simulink model "Extended_Kalman_Filter_Simulink_Example"  (R2024b)
settings: Solver=VariableStepAuto  StartTime=0.0  StopTime=20  RelTol=1e-3
libraries: simulink x5
settings Model: Creator=mulusoy  LastModifiedBy=fouca
settings SolverCC: AlgebraicLoopSolver=TrustRegion
settings DataIOCC: ReturnWorkspaceOutputs=off
settings OptimizationCC: BlockReduction=off  DefaultParameterBehavior=Inlined  ExpressionFolding=off  PassReuseOutputArgsAs=Individual arguments  EfficientTunableParamExpr=on
settings DebuggingCC: ParameterTunabilityLossMsg=error  ArithmeticOperatorsInVariantConditions=warning
settings ModelReferenceCC: EnableRefExpFcnMdlSchedulingChecks=on
settings SFSimCC: SimUseLocalCustomCode=off  MATLABDynamicMemAlloc=off  CustomCodeUndefinedFunction=UseInterfaceOnly
settings RTWCC: Description=Embedded Coder  SystemTargetFile=ert.tlc  GenCodeOnly=on  TemplateMakefile=ert_default_tmf  GenerateReport=on  RTWUseLocalCustomCode=off  IncludeHyperlinkInReport=on  LaunchReport=on  GenerateTraceInfo=on  GenerateTraceReport=on  GenerateTraceReportSl=on  GenerateTraceReportSf=on  GenerateTraceReportEml=on  GPUComputeCapability=3.5
settings CodeAppCC: ForceParamTrailComments=on  IgnoreCustomStorageClasses=off  OperatorAnnotations=on  SimulinkDataObjDesc=on  SFDataObjDesc=on  MATLABFcnDesc=on  InsertBlockDesc=on  StateflowObjectComments=on  MATLABSourceComments=on  EnableCustomComments=on  InlinedPrmAccess=Macros  ReqsInCode=on
settings ERTTargetCC: TargetLangStandard=C99 (ISO)  GenerateSampleERTMain=on  ERTCustomFileTemplate=example_file_process.tlc  ConvertIfToSwitch=off  DynamicArrayContainerType=coder::array
settings DiagnosticsConfigSet: SimMechanicsInvalidVisualProperty=none  SimMechanicsCrossSectionNullEdge=none  SimMechanicsUnconnectedFramePorts=none  SimMechanicsUnconnectedGeometryPorts=none  SimMechanicsRedundantBlock=none  SimMechanicsConflictingReferenceFrames=none  SimMechanicsUnsatisfiedHighPriorityTargets=none
settings ExplorerConfigSet: InternalSimMechanicsExplorerSettings="<ExplorerConfiguration><canonicalview>aerospace</canonicalview><AnimationSetting><BasePlaybackSpeed>1.0</BasePlaybackSpeed><PlaybackSpeedFactor>1.0</PlaybackSpeedFactor></AnimationSetting><TilePanel><TileInfo><Tiles Columns=\"1\" Count=\"1\" Rows=\"1\"><Column Weight=\"1\"/><Row Weight=\"1\"/><Tile Height=\"1\" Width=\"1\" X=\"0\" Y=\"0\"/></Tiles></TileInfo><SceneInfo><SceneViewer><BGColor><R>0.60000002384185791</R><G>0.60000002384185791</G><B>0.60000002384185791</B></BGColor><Camera><DoPerspective>off</DoPerspective><Position><X>-3.66024810460885419e-09</X><Y>-0.263498918054518638</Y><Z>1.00000000158182067</Z></Position><Center><X>-3.66024810460885419e-09</X><Y>-0.263498918054518638</Y><Z>1.58182067444556651e-09</Z></Center><Up><X>0</X><Y>1</Y><Z>0</Z></Up><ViewLimDist>1</ViewLimDist><YLim>0.297153875529766076</YLim><XLim>0.39010476366144331</XLim></Camera></SceneViewer></SceneInfo></TilePanel><MechEditorPanel><Cameras/><GfxPanelCameraMap/><VideoCreator><PlaybackSpeedRatio>1.0</PlaybackSpeedRatio><FrameRate>30</FrameRate><VideoFormat>Motion JPEG AVI</VideoFormat><FrameSize>auto</FrameSize></VideoCreator></MechEditorPanel></ExplorerConfiguration>"

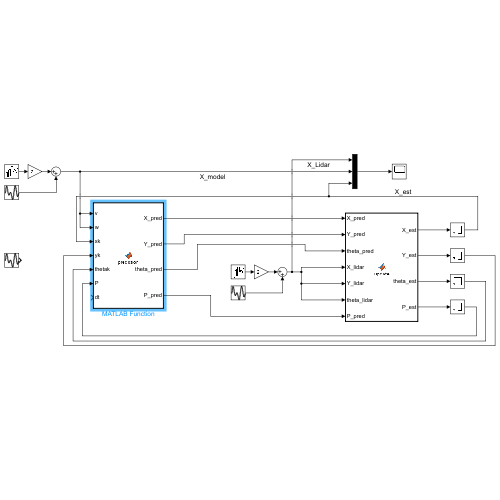
[thumbnail: Simulink's stored preview of the top-level diagram]
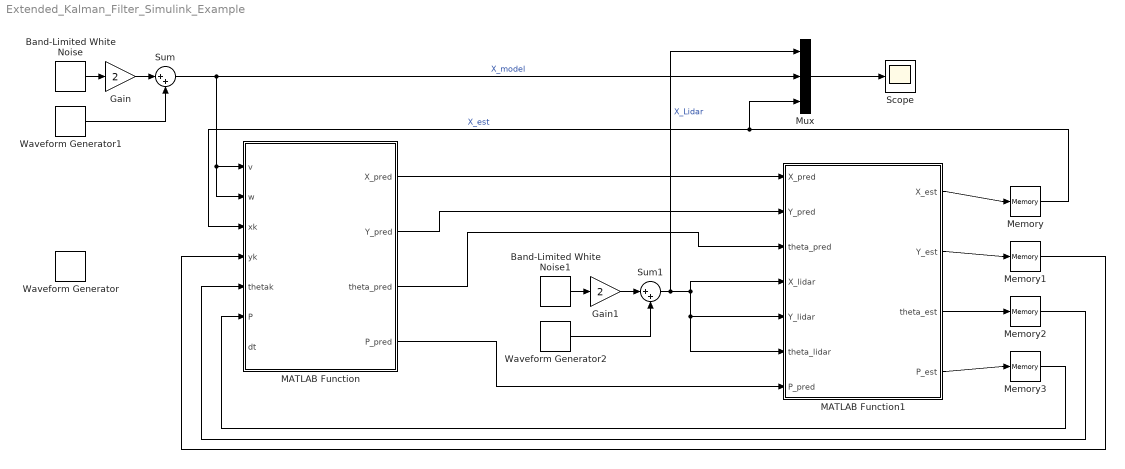
== system Extended_Kalman_Filter_Simulink_Example ==
  Band-Limited White Noise : simulink/Sources/Band-Limited White Noise  Cov=[0.1]  Ts=0.1  seed=[23341]
  Band-Limited White Noise1 : simulink/Sources/Band-Limited White Noise  Cov=[0.1]  Ts=0.1  seed=[23341]
  Gain : Gain  Gain=2
  Gain1 : Gain  Gain=2
  MATLAB Function : MATLAB Function  TreatAsAtomicUnit=on
  MATLAB Function1 : MATLAB Function  TreatAsAtomicUnit=on
  Memory{,1..3} (4 alike) : Memory
  Mux : Mux  Inputs=3
  Scope : Scope
  Sum : Sum  Inputs=|++
  Sum1 : Sum  Inputs=|++
  Waveform Generator : simulink/Sources/Waveform Generator  OutMin=[]  OutMax=[]  OutDataTypeStr=double  SelectedSignal=1  Signals=sin()#  BlockNames=MultiportSwitch_64de44b0bc4e432#MultiportSwitch_e4664bebc71b4e7  SampleTime=0.1
  Waveform Generator1 : simulink/Sources/Waveform Generator  OutMin=[]  OutMax=[]  OutDataTypeStr=double  SelectedSignal=1  Signals=10*sin()#  BlockNames=MultiportSwitch_8758bd99aa354f9#MultiportSwitch_3944adbdd2c94b6  SampleTime=0.1
  Waveform Generator2 : simulink/Sources/Waveform Generator  OutMin=[]  OutMax=[]  OutDataTypeStr=double  SelectedSignal=1  Signals=4*sin()#  BlockNames=MultiportSwitch_75d6421b91b44ed#MultiportSwitch_4d6c01110f4e42d  SampleTime=0.1
  wires:
  MATLAB Function/2(Y_pred) -> MATLAB Function1/2(Y_pred)
  MATLAB Function/3(theta_pred) -> MATLAB Function1/3(theta_pred)
  MATLAB Function/4(P_pred) -> MATLAB Function1/7(P_pred)
  MATLAB Function1/1(X_est) -> Memory/1
  MATLAB Function1/2(Y_est) -> Memory1/1
  MATLAB Function1/3(theta_est) -> Memory2/1
  MATLAB Function1/4(P_est) -> Memory3/1
  Memory3/1 -> MATLAB Function/6(P)
  Memory2/1 -> MATLAB Function/5(thetak)
  Memory1/1 -> MATLAB Function/4(yk)
  Memory/1 -> Mux/3, MATLAB Function/3(xk)  "X_est"
  Waveform Generator1/1 -> Sum/2
  Band-Limited White Noise/1 -> Gain/1
  Gain/1 -> Sum/1
  Sum/1 -> MATLAB Function/2(w), MATLAB Function/1(v), Mux/2  "X_model"
  Sum1/1 -> Mux/1, MATLAB Function1/6(theta_lidar), MATLAB Function1/5(Y_lidar), MATLAB Function1/4(X_lidar)  "X_Lidar"
  Waveform Generator2/1 -> Sum1/2
  Gain1/1 -> Sum1/1
  Band-Limited White Noise1/1 -> Gain1/1
  Mux/1 -> Scope/1
  MATLAB Function/1(X_pred) -> MATLAB Function1/1(X_pred)

== matlab function Extended_Kalman_Filter_Simulink_Example/MATLAB Function1 ==
  data: X_pred input; X_est output; Y_pred input; theta_pred input; X_lidar input; Y_lidar input; theta_lidar input; P_pred input; Y_est output; theta_est output; P_est output
function [X_est, Y_est, theta_est, P_est] = update(X_pred, Y_pred, theta_pred, X_lidar, Y_lidar, theta_lidar, P_pred)
    % 1. VECTEURS D'ÉTAT ET DE MESURE
    x_p = [X_pred; Y_pred; theta_pred];
    z = [X_lidar; Y_lidar; theta_lidar];

    % 2. MODÈLE D'OBSERVATION (H)
    % Puisque le LIDAR mesure directement x, y et theta, H est l'identité
    H = eye(3);

    % 3. MATRICE DE BRUIT DE MESURE (R)
    % Plus ces valeurs sont faibles, plus le filtre fera confiance au LIDAR
    % (À ajuster selon la précision de votre LIDAR)
    r_dist = 0.05; % Incertitude en mètres
    r_ang  = 0.02; % Incertitude en radians
    R = diag([r_dist, r_dist, r_ang]);

    % 4. CALCUL DU GAIN DE KALMAN (K)
    % S est la covariance de l'innovation
    S = H * P_pred * H' + R;
    K = P_pred * H' / S;

    % 5. CALCUL DE L'INNOVATION (Erreur entre LIDAR et Prédiction)
    innovation = z - (H * x_p);

    % --- TRÈS IMPORTANT : Normalisation de l'erreur d'angle ---
    % Empêche le filtre de paniquer si le LIDAR dit 179° et le modèle 181° (-179°)
    innovation(3) = atan2(sin(innovation(3)), cos(innovation(3)));

    % 6. MISE À JOUR DE L'ÉTAT ET DE LA COVARIANCE
    x_corrected = x_p + K * innovation;
    P_corrected = (eye(3) - K * H) * P_pred;

    % 7. ASSIGNATION DES SORTIES
    X_est = x_corrected(1);
    Y_est = x_corrected(2);
    theta_est = atan2(sin(x_corrected(3)), cos(x_corrected(3)));
    P_est = P_corrected;
end

== matlab function Extended_Kalman_Filter_Simulink_Example/MATLAB Function ==
  data: v input; X_pred output; w input; xk input; yk input; thetak input; P input; dt input; Y_pred output; theta_pred output; P_pred output
function [X_pred, Y_pred, theta_pred, P_pred] = prediction(v, w, xk, yk, thetak, P, dt)
    % Vecteur d'état actuel
    X = [xk; yk; thetak];
    
    % 1. MODÈLE D'ÉTAT (Cinématique du QBot)
    % On calcule la prédiction basée sur les vitesses v (linéaire) et w (angulaire)
    X_next = X + [v * cos(thetak) * dt;
                  v * sin(thetak) * dt;
                  w * dt];
    
    % Extraction des sorties
    X_pred     = X_next(1);
    Y_pred     = X_next(2);
    theta_pred = atan2(sin(X_next(3)), cos(X_next(3))); % Normalisation d'angle (-pi à pi)

    % 2. LINÉARISATION (Calcul de la Jacobienne F)
    % f est la dérivée de l'équation d'état par rapport à x, y et theta
    F = [1, 0, -v * sin(thetak) * dt;
         0, 1,  v * cos(thetak) * dt;
         0, 0,  1];

    % 3. BRUIT DE MODÈLE (Matrice Q)
    % Plus ces valeurs sont élevées, moins on fait confiance au modèle théorique
    % À ajuster selon les glissements des roues du QBot
    q_x = 0.01; 
    q_y = 0.01;
    q_theta = 0.02;
    Q = diag([q_x, q_y, q_theta]);

    % 4. PRÉDICTION DE LA COVARIANCE
    % On propage l'incertitude P_pred = F*P*F' + Q
    P_pred = F * P * F' + Q;
end
